simulink model "Demo_V2X_RoadWorks_cs"  (R2014b)
settings: Solver=ode5  SolverMode=SingleTasking  StartTime=0.0  StopTime=18  FixedStep=1/100  RelTol=1e-3
PreLoadFcn:
  | mbxruntime.callbacks.PreLoadFcn(bdroot);
  | check_NUTS_defined;
  | 
  | assignin('base',['model_closed_' bdroot],false);
PostLoadFcn:
  | mbxruntime.callbacks.PostLoadFcn(bdroot);
InitFcn:
  | mbxruntime.callbacks.InitFcn(bdroot);
StartFcn:
  | mbxruntime.callbacks.StartFcn(bdroot);
StopFcn:
  | mbxruntime.callbacks.StopFcn(bdroot);
model workspace: external: MAT-File .\Demo_V2X_RoadWorks_cs_hws.mat (data not in the file)
undefined symbols (not defined in the file or in its folder): InitializeBus, mbxruntime, Newton, Raphson, tabledata
undefined symbols (not defined in the file): Demo_V2X_RoadWorks_cs_002408181c311178, Demo_V2X_RoadWorks_cs_02afd40c5576fd79, Demo_V2X_RoadWorks_cs_09062d95c4976b80, Demo_V2X_RoadWorks_cs_0ad60e46608f1bfe, Demo_V2X_RoadWorks_cs_0b386a01b2cd5e8d, Demo_V2X_RoadWorks_cs_0d795afaa024d2ee, Demo_V2X_RoadWorks_cs_104085e65c337077, Demo_V2X_RoadWorks_cs_126564f7b2997a49, Demo_V2X_RoadWorks_cs_15e6e2595e8bf329, Demo_V2X_RoadWorks_cs_16adfea7655bce18, Demo_V2X_RoadWorks_cs_18ab2686f8449f50, Demo_V2X_RoadWorks_cs_1c28437def32f9f6, Demo_V2X_RoadWorks_cs_1d541c73c3d8f25b, Demo_V2X_RoadWorks_cs_1fb1f994fe012d27, Demo_V2X_RoadWorks_cs_20c117b9827230b9, Demo_V2X_RoadWorks_cs_220b1226a84e3b37, Demo_V2X_RoadWorks_cs_24814049c8ab2e18, Demo_V2X_RoadWorks_cs_24a281220a6492a7, Demo_V2X_RoadWorks_cs_279aea126b4236ad, Demo_V2X_RoadWorks_cs_28eadd0b23e572db, Demo_V2X_RoadWorks_cs_291fe7210f9ba434, Demo_V2X_RoadWorks_cs_2fd90504f8814746, Demo_V2X_RoadWorks_cs_33c1737bfc1c651f, Demo_V2X_RoadWorks_cs_388e22d5b1056b8f, Demo_V2X_RoadWorks_cs_3e3a415e868663e7, Demo_V2X_RoadWorks_cs_45759eb0c1816b1e, Demo_V2X_RoadWorks_cs_45f301cf6c396570, Demo_V2X_RoadWorks_cs_47686124f5151dea, Demo_V2X_RoadWorks_cs_487931e8a8cef1d6, Demo_V2X_RoadWorks_cs_54cb5626dca53ab7, Demo_V2X_RoadWorks_cs_56c0a253fe7e7ec0, Demo_V2X_RoadWorks_cs_5921488c0ba4168e, Demo_V2X_RoadWorks_cs_5ca0c70551eea1b3, Demo_V2X_RoadWorks_cs_5cc6ddb60eb17926, Demo_V2X_RoadWorks_cs_5dda33a127b53dd9, Demo_V2X_RoadWorks_cs_60729aca19e3b8ea, Demo_V2X_RoadWorks_cs_61616eaaf58ec115, Demo_V2X_RoadWorks_cs_63af626c9fae5224, Demo_V2X_RoadWorks_cs_649c6af7b111a61f, Demo_V2X_RoadWorks_cs_64e2df335ac415c1, Demo_V2X_RoadWorks_cs_6530f1ae727e39fe, Demo_V2X_RoadWorks_cs_6837be8d052ff1e3, Demo_V2X_RoadWorks_cs_6e8b51a123f1a201, Demo_V2X_RoadWorks_cs_6f4ec518a68cacb3, Demo_V2X_RoadWorks_cs_74dac4a6b9859226, Demo_V2X_RoadWorks_cs_75671d8cae67d5b6, Demo_V2X_RoadWorks_cs_756d40a88ae84d39, Demo_V2X_RoadWorks_cs_77c7cbc4fa1cdaa5, Demo_V2X_RoadWorks_cs_7b9fbc44403bb8f3, Demo_V2X_RoadWorks_cs_7c118b74c8d14c00, Demo_V2X_RoadWorks_cs_7c4a172761f05beb, Demo_V2X_RoadWorks_cs_80b7a78efe24d5f1, Demo_V2X_RoadWorks_cs_82d65efce1f7c4ea, Demo_V2X_RoadWorks_cs_8be5dc2565229ce9, Demo_V2X_RoadWorks_cs_8dc36f0ab6cec640, Demo_V2X_RoadWorks_cs_91305dd1362bb00d, Demo_V2X_RoadWorks_cs_929c2ffed1faf33f, Demo_V2X_RoadWorks_cs_95615bcbc0d062f1, Demo_V2X_RoadWorks_cs_99a6391a40f894df, Demo_V2X_RoadWorks_cs_9caa19175765ea5d ... (+52)
libraries: PreScanSimulinkLibrary x34, simulink_extras x15, simulink x6
(part 5 of 16)

== system Demo_V2X_RoadWorks_cs/SELF_Male_Regular_BendingOver_1 ==
  Sensor : S-Function  FunctionName=sfun_SelfSensor  Parameters=UniqueID, TimeStep  EnableBusSupport=off  mask(PreScan Source Block: SELF){UniqueID=4029, TimeStep=1/100}
      mask prompts: UniqueID "Auto-Assigned: Unique ID"; TimeStep "Auto-Assigned: Upload Period [s]"
      mask help:
      | The SELF port shows (state) information of the actor itself. The outputs are position in the experiment's axis system and the GPS coordinates, and the object's absolute velocity and compass heading.
      |
      | For more information, please click Help.
      mask Help: eval('openHelp(462)')
      mask Display: image(imread('GPS.png'))
  SELF_Male_Regular_BendingOver_1 : Outport  Tag=outport/SelfPort  OutDataTypeStr=Bus: PRESCAN_SELFSENSORDATA  PortDimensions=1  SampleTime=1/100
  wires:
  Sensor/1 -> SELF_Male_Regular_BendingOver_1/1

== system Demo_V2X_RoadWorks_cs/SELF_Male_Regular_LeaningBack_1 ==
  Sensor : S-Function  FunctionName=sfun_SelfSensor  Parameters=UniqueID, TimeStep  EnableBusSupport=off  mask(PreScan Source Block: SELF){UniqueID=4031, TimeStep=1/100}
      mask prompts: UniqueID "Auto-Assigned: Unique ID"; TimeStep "Auto-Assigned: Upload Period [s]"
      mask help:
      | The SELF port shows (state) information of the actor itself. The outputs are position in the experiment's axis system and the GPS coordinates, and the object's absolute velocity and compass heading.
      |
      | For more information, please click Help.
      mask Help: eval('openHelp(462)')
      mask Display: image(imread('GPS.png'))
  SELF_Male_Regular_LeaningBack_1 : Outport  Tag=outport/SelfPort  OutDataTypeStr=Bus: PRESCAN_SELFSENSORDATA  PortDimensions=1  SampleTime=1/100
  wires:
  Sensor/1 -> SELF_Male_Regular_LeaningBack_1/1

== system Demo_V2X_RoadWorks_cs/SELF_Male_Regular_LeaningBack_2 ==
  Sensor : S-Function  FunctionName=sfun_SelfSensor  Parameters=UniqueID, TimeStep  EnableBusSupport=off  mask(PreScan Source Block: SELF){UniqueID=4032, TimeStep=1/100}
      mask prompts: UniqueID "Auto-Assigned: Unique ID"; TimeStep "Auto-Assigned: Upload Period [s]"
      mask help:
      | The SELF port shows (state) information of the actor itself. The outputs are position in the experiment's axis system and the GPS coordinates, and the object's absolute velocity and compass heading.
      |
      | For more information, please click Help.
      mask Help: eval('openHelp(462)')
      mask Display: image(imread('GPS.png'))
  SELF_Male_Regular_LeaningBack_2 : Outport  Tag=outport/SelfPort  OutDataTypeStr=Bus: PRESCAN_SELFSENSORDATA  PortDimensions=1  SampleTime=1/100
  wires:
  Sensor/1 -> SELF_Male_Regular_LeaningBack_2/1

== system Demo_V2X_RoadWorks_cs/SELF_Male_Regular_Leaning_1 ==
  Sensor : S-Function  FunctionName=sfun_SelfSensor  Parameters=UniqueID, TimeStep  EnableBusSupport=off  mask(PreScan Source Block: SELF){UniqueID=4030, TimeStep=1/100}
      mask prompts: UniqueID "Auto-Assigned: Unique ID"; TimeStep "Auto-Assigned: Upload Period [s]"
      mask help:
      | The SELF port shows (state) information of the actor itself. The outputs are position in the experiment's axis system and the GPS coordinates, and the object's absolute velocity and compass heading.
      |
      | For more information, please click Help.
      mask Help: eval('openHelp(462)')
      mask Display: image(imread('GPS.png'))
  SELF_Male_Regular_Leaning_1 : Outport  Tag=outport/SelfPort  OutDataTypeStr=Bus: PRESCAN_SELFSENSORDATA  PortDimensions=1  SampleTime=1/100
  wires:
  Sensor/1 -> SELF_Male_Regular_Leaning_1/1

== system Demo_V2X_RoadWorks_cs/SELF_Male_Regular_LyingDown_1 ==
  Sensor : S-Function  FunctionName=sfun_SelfSensor  Parameters=UniqueID, TimeStep  EnableBusSupport=off  mask(PreScan Source Block: SELF){UniqueID=4028, TimeStep=1/100}
      mask prompts: UniqueID "Auto-Assigned: Unique ID"; TimeStep "Auto-Assigned: Upload Period [s]"
      mask help:
      | The SELF port shows (state) information of the actor itself. The outputs are position in the experiment's axis system and the GPS coordinates, and the object's absolute velocity and compass heading.
      |
      | For more information, please click Help.
      mask Help: eval('openHelp(462)')
      mask Display: image(imread('GPS.png'))
  SELF_Male_Regular_LyingDown_1 : Outport  Tag=outport/SelfPort  OutDataTypeStr=Bus: PRESCAN_SELFSENSORDATA  PortDimensions=1  SampleTime=1/100
  wires:
  Sensor/1 -> SELF_Male_Regular_LyingDown_1/1

== system Demo_V2X_RoadWorks_cs/SELF_Mazda_RX8_1 ==
  Sensor : S-Function  FunctionName=sfun_SelfSensor  Parameters=UniqueID, TimeStep  EnableBusSupport=off  mask(PreScan Source Block: SELF){UniqueID=3607, TimeStep=1/100}
      mask prompts: UniqueID "Auto-Assigned: Unique ID"; TimeStep "Auto-Assigned: Upload Period [s]"
      mask help:
      | The SELF port shows (state) information of the actor itself. The outputs are position in the experiment's axis system and the GPS coordinates, and the object's absolute velocity and compass heading.
      |
      | For more information, please click Help.
      mask Help: eval('openHelp(462)')
      mask Display: image(imread('GPS.png'))
  SELF_Mazda_RX8_1 : Outport  Tag=outport/SelfPort  OutDataTypeStr=Bus: PRESCAN_SELFSENSORDATA  PortDimensions=1  SampleTime=1/100
  wires:
  Sensor/1 -> SELF_Mazda_RX8_1/1

== system Demo_V2X_RoadWorks_cs/SELF_Nissan_Cabstar_1 ==
  Sensor : S-Function  FunctionName=sfun_SelfSensor  Parameters=UniqueID, TimeStep  EnableBusSupport=off  mask(PreScan Source Block: SELF){UniqueID=3606, TimeStep=1/100}
      mask prompts: UniqueID "Auto-Assigned: Unique ID"; TimeStep "Auto-Assigned: Upload Period [s]"
      mask help:
      | The SELF port shows (state) information of the actor itself. The outputs are position in the experiment's axis system and the GPS coordinates, and the object's absolute velocity and compass heading.
      |
      | For more information, please click Help.
      mask Help: eval('openHelp(462)')
      mask Display: image(imread('GPS.png'))
  SELF_Nissan_Cabstar_1 : Outport  Tag=outport/SelfPort  OutDataTypeStr=Bus: PRESCAN_SELFSENSORDATA  PortDimensions=1  SampleTime=1/100
  wires:
  Sensor/1 -> SELF_Nissan_Cabstar_1/1

== system Demo_V2X_RoadWorks_cs/SELF_Sphere_1 ==
  Sensor : S-Function  FunctionName=sfun_SelfSensor  Parameters=UniqueID, TimeStep  EnableBusSupport=off  mask(PreScan Source Block: SELF){UniqueID=3615, TimeStep=1/100}
      mask prompts: UniqueID "Auto-Assigned: Unique ID"; TimeStep "Auto-Assigned: Upload Period [s]"
      mask help:
      | The SELF port shows (state) information of the actor itself. The outputs are position in the experiment's axis system and the GPS coordinates, and the object's absolute velocity and compass heading.
      |
      | For more information, please click Help.
      mask Help: eval('openHelp(462)')
      mask Display: image(imread('GPS.png'))
  SELF_Sphere_1 : Outport  Tag=outport/SelfPort  OutDataTypeStr=Bus: PRESCAN_SELFSENSORDATA  PortDimensions=1  SampleTime=1/100
  wires:
  Sensor/1 -> SELF_Sphere_1/1

== system Demo_V2X_RoadWorks_cs/SELF_Toyota_Previa_1 ==
  Sensor : S-Function  FunctionName=sfun_SelfSensor  Parameters=UniqueID, TimeStep  EnableBusSupport=off  mask(PreScan Source Block: SELF){UniqueID=3608, TimeStep=1/100}
      mask prompts: UniqueID "Auto-Assigned: Unique ID"; TimeStep "Auto-Assigned: Upload Period [s]"
      mask help:
      | The SELF port shows (state) information of the actor itself. The outputs are position in the experiment's axis system and the GPS coordinates, and the object's absolute velocity and compass heading.
      |
      | For more information, please click Help.
      mask Help: eval('openHelp(462)')
      mask Display: image(imread('GPS.png'))
  SELF_Toyota_Previa_1 : Outport  Tag=outport/SelfPort  OutDataTypeStr=Bus: PRESCAN_SELFSENSORDATA  PortDimensions=1  SampleTime=1/100
  wires:
  Sensor/1 -> SELF_Toyota_Previa_1/1

== system Demo_V2X_RoadWorks_cs/SELF_Toyota_Yaris_1 ==
  Sensor : S-Function  FunctionName=sfun_SelfSensor  Parameters=UniqueID, TimeStep  EnableBusSupport=off  mask(PreScan Source Block: SELF){UniqueID=3534, TimeStep=1/100}
      mask prompts: UniqueID "Auto-Assigned: Unique ID"; TimeStep "Auto-Assigned: Upload Period [s]"
      mask help:
      | The SELF port shows (state) information of the actor itself. The outputs are position in the experiment's axis system and the GPS coordinates, and the object's absolute velocity and compass heading.
      |
      | For more information, please click Help.
      mask Help: eval('openHelp(462)')
      mask Display: image(imread('GPS.png'))
  SELF_Toyota_Yaris_1 : Outport  Tag=outport/SelfPort  OutDataTypeStr=Bus: PRESCAN_SELFSENSORDATA  PortDimensions=1  SampleTime=1/100
  wires:
  Sensor/1 -> SELF_Toyota_Yaris_1/1

== system Demo_V2X_RoadWorks_cs/STATE_Actros_1860_1_bus ==
  STATE_Actros_1860_1_bus : Inport  Tag=inport/StatePort  OutDataTypeStr=Bus: PRESCAN_STATEACTUATORDATA  PortDimensions=1  SampleTime=1/100  BusOutputAsStruct=on
  Actuator : S-Function  FunctionName=sfun_StateActuator  Parameters=UniqueID, TimeStep  EnableBusSupport=off  mask(PreScan Sink Block: State){UniqueID=3711, TimeStep=1/100}
      mask prompts: UniqueID "Auto-Assigned: Unique ID"; TimeStep "Auto-Assigned: Upload Period [s]"
      mask help:
      | The Actor State contains a vector signal of size (9x1), containing the following signals:
      |
      | -  Position    	(x,y,z)             	[m]
      | -  Velocity    	(vx,vy,vz)         	[m/s]
      | -  Angles       	(Roll, Pitch, Yaw)	[rad]
      |
      | The Actor state is defined in the global axis system.
      | The state is superponed on the Initial position defined in the GUI.
      |
      | For more information, please click Help.
      mask Help: eval('openHelp(222)')
      mask Display: image(imread('State.png'))
  wires:
  STATE_Actros_1860_1_bus/1 -> Actuator/1

== system Demo_V2X_RoadWorks_cs/STATE_Actros_2541_1_bus ==
  STATE_Actros_2541_1_bus : Inport  Tag=inport/StatePort  OutDataTypeStr=Bus: PRESCAN_STATEACTUATORDATA  PortDimensions=1  SampleTime=1/100  BusOutputAsStruct=on
  Actuator : S-Function  FunctionName=sfun_StateActuator  Parameters=UniqueID, TimeStep  EnableBusSupport=off  mask(PreScan Sink Block: State){UniqueID=3609, TimeStep=1/100}
      mask prompts: UniqueID "Auto-Assigned: Unique ID"; TimeStep "Auto-Assigned: Upload Period [s]"
      mask help:
      | The Actor State contains a vector signal of size (9x1), containing the following signals:
      |
      | -  Position    	(x,y,z)             	[m]
      | -  Velocity    	(vx,vy,vz)         	[m/s]
      | -  Angles       	(Roll, Pitch, Yaw)	[rad]
      |
      | The Actor state is defined in the global axis system.
      | The state is superponed on the Initial position defined in the GUI.
      |
      | For more information, please click Help.
      mask Help: eval('openHelp(222)')
      mask Display: image(imread('State.png'))
  wires:
  STATE_Actros_2541_1_bus/1 -> Actuator/1

== system Demo_V2X_RoadWorks_cs/STATE_Audi_A8_1_bus ==
  STATE_Audi_A8_1_bus : Inport  Tag=inport/StatePort  OutDataTypeStr=Bus: PRESCAN_STATEACTUATORDATA  PortDimensions=1  SampleTime=1/100  BusOutputAsStruct=on
  Actuator : S-Function  FunctionName=sfun_StateActuator  Parameters=UniqueID, TimeStep  EnableBusSupport=off  mask(PreScan Sink Block: State){UniqueID=1227, TimeStep=1/100}
      mask prompts: UniqueID "Auto-Assigned: Unique ID"; TimeStep "Auto-Assigned: Upload Period [s]"
      mask help:
      | The Actor State contains a vector signal of size (9x1), containing the following signals:
      |
      | -  Position    	(x,y,z)             	[m]
      | -  Velocity    	(vx,vy,vz)         	[m/s]
      | -  Angles       	(Roll, Pitch, Yaw)	[rad]
      |
      | The Actor state is defined in the global axis system.
      | The state is superponed on the Initial position defined in the GUI.
      |
      | For more information, please click Help.
      mask Help: eval('openHelp(222)')
      mask Display: image(imread('State.png'))
  wires:
  STATE_Audi_A8_1_bus/1 -> Actuator/1

== system Demo_V2X_RoadWorks_cs/STATE_BMW_X5_1_bus ==
  STATE_BMW_X5_1_bus : Inport  Tag=inport/StatePort  OutDataTypeStr=Bus: PRESCAN_STATEACTUATORDATA  PortDimensions=1  SampleTime=1/100  BusOutputAsStruct=on
  Actuator : S-Function  FunctionName=sfun_StateActuator  Parameters=UniqueID, TimeStep  EnableBusSupport=off  mask(PreScan Sink Block: State){UniqueID=3531, TimeStep=1/100}
      mask prompts: UniqueID "Auto-Assigned: Unique ID"; TimeStep "Auto-Assigned: Upload Period [s]"
      mask help:
      | The Actor State contains a vector signal of size (9x1), containing the following signals:
      |
      | -  Position    	(x,y,z)             	[m]
      | -  Velocity    	(vx,vy,vz)         	[m/s]
      | -  Angles       	(Roll, Pitch, Yaw)	[rad]
      |
      | The Actor state is defined in the global axis system.
      | The state is superponed on the Initial position defined in the GUI.
      |
      | For more information, please click Help.
      mask Help: eval('openHelp(222)')
      mask Display: image(imread('State.png'))
  wires:
  STATE_BMW_X5_1_bus/1 -> Actuator/1

== system Demo_V2X_RoadWorks_cs/STATE_CarTrailer_SingleAxle_1_bus ==
  STATE_CarTrailer_SingleAxle_1_bus : Inport  Tag=inport/StatePort  OutDataTypeStr=Bus: PRESCAN_STATEACTUATORDATA  PortDimensions=1  SampleTime=1/100  BusOutputAsStruct=on
  Actuator : S-Function  FunctionName=sfun_StateActuator  Parameters=UniqueID, TimeStep  EnableBusSupport=off  mask(PreScan Sink Block: State){UniqueID=4026, TimeStep=1/100}
      mask prompts: UniqueID "Auto-Assigned: Unique ID"; TimeStep "Auto-Assigned: Upload Period [s]"
      mask help:
      | The Actor State contains a vector signal of size (9x1), containing the following signals:
      |
      | -  Position    	(x,y,z)             	[m]
      | -  Velocity    	(vx,vy,vz)         	[m/s]
      | -  Angles       	(Roll, Pitch, Yaw)	[rad]
      |
      | The Actor state is defined in the global axis system.
      | The state is superponed on the Initial position defined in the GUI.
      |
      | For more information, please click Help.
      mask Help: eval('openHelp(222)')
      mask Display: image(imread('State.png'))
  wires:
  STATE_CarTrailer_SingleAxle_1_bus/1 -> Actuator/1

== system Demo_V2X_RoadWorks_cs/STATE_ChessPlaneBox_1_bus ==
  STATE_ChessPlaneBox_1_bus : Inport  Tag=inport/StatePort  OutDataTypeStr=Bus: PRESCAN_STATEACTUATORDATA  PortDimensions=1  SampleTime=1/100  BusOutputAsStruct=on
  Actuator : S-Function  FunctionName=sfun_StateActuator  Parameters=UniqueID, TimeStep  EnableBusSupport=off  mask(PreScan Sink Block: State){UniqueID=4034, TimeStep=1/100}
      mask prompts: UniqueID "Auto-Assigned: Unique ID"; TimeStep "Auto-Assigned: Upload Period [s]"
      mask help:
      | The Actor State contains a vector signal of size (9x1), containing the following signals:
      |
      | -  Position    	(x,y,z)             	[m]
      | -  Velocity    	(vx,vy,vz)         	[m/s]
      | -  Angles       	(Roll, Pitch, Yaw)	[rad]
      |
      | The Actor state is defined in the global axis system.
      | The state is superponed on the Initial position defined in the GUI.
      |
      | For more information, please click Help.
      mask Help: eval('openHelp(222)')
      mask Display: image(imread('State.png'))
  wires:
  STATE_ChessPlaneBox_1_bus/1 -> Actuator/1

== system Demo_V2X_RoadWorks_cs/STATE_Citroen_C3_1_bus ==
  STATE_Citroen_C3_1_bus : Inport  Tag=inport/StatePort  OutDataTypeStr=Bus: PRESCAN_STATEACTUATORDATA  PortDimensions=1  SampleTime=1/100  BusOutputAsStruct=on
  Actuator : S-Function  FunctionName=sfun_StateActuator  Parameters=UniqueID, TimeStep  EnableBusSupport=off  mask(PreScan Sink Block: State){UniqueID=3533, TimeStep=1/100}
      mask prompts: UniqueID "Auto-Assigned: Unique ID"; TimeStep "Auto-Assigned: Upload Period [s]"
      mask help:
      | The Actor State contains a vector signal of size (9x1), containing the following signals:
      |
      | -  Position    	(x,y,z)             	[m]
      | -  Velocity    	(vx,vy,vz)         	[m/s]
      | -  Angles       	(Roll, Pitch, Yaw)	[rad]
      |
      | The Actor state is defined in the global axis system.
      | The state is superponed on the Initial position defined in the GUI.
      |
      | For more information, please click Help.
      mask Help: eval('openHelp(222)')
      mask Display: image(imread('State.png'))
  wires:
  STATE_Citroen_C3_1_bus/1 -> Actuator/1

== system Demo_V2X_RoadWorks_cs/STATE_Fiat_Bravo_1_bus ==
  STATE_Fiat_Bravo_1_bus : Inport  Tag=inport/StatePort  OutDataTypeStr=Bus: PRESCAN_STATEACTUATORDATA  PortDimensions=1  SampleTime=1/100  BusOutputAsStruct=on
  Actuator : S-Function  FunctionName=sfun_StateActuator  Parameters=UniqueID, TimeStep  EnableBusSupport=off  mask(PreScan Sink Block: State){UniqueID=3535, TimeStep=1/100}
      mask prompts: UniqueID "Auto-Assigned: Unique ID"; TimeStep "Auto-Assigned: Upload Period [s]"
      mask help:
      | The Actor State contains a vector signal of size (9x1), containing the following signals:
      |
      | -  Position    	(x,y,z)             	[m]
      | -  Velocity    	(vx,vy,vz)         	[m/s]
      | -  Angles       	(Roll, Pitch, Yaw)	[rad]
      |
      | The Actor state is defined in the global axis system.
      | The state is superponed on the Initial position defined in the GUI.
      |
      | For more information, please click Help.
      mask Help: eval('openHelp(222)')
      mask Display: image(imread('State.png'))
  wires:
  STATE_Fiat_Bravo_1_bus/1 -> Actuator/1

== system Demo_V2X_RoadWorks_cs/STATE_Ford_FocusWagon_1_bus ==
  STATE_Ford_FocusWagon_1_bus : Inport  Tag=inport/StatePort  OutDataTypeStr=Bus: PRESCAN_STATEACTUATORDATA  PortDimensions=1  SampleTime=1/100  BusOutputAsStruct=on
  Actuator : S-Function  FunctionName=sfun_StateActuator  Parameters=UniqueID, TimeStep  EnableBusSupport=off  mask(PreScan Sink Block: State){UniqueID=3532, TimeStep=1/100}
      mask prompts: UniqueID "Auto-Assigned: Unique ID"; TimeStep "Auto-Assigned: Upload Period [s]"
      mask help:
      | The Actor State contains a vector signal of size (9x1), containing the following signals:
      |
      | -  Position    	(x,y,z)             	[m]
      | -  Velocity    	(vx,vy,vz)         	[m/s]
      | -  Angles       	(Roll, Pitch, Yaw)	[rad]
      |
      | The Actor state is defined in the global axis system.
      | The state is superponed on the Initial position defined in the GUI.
      |
      | For more information, please click Help.
      mask Help: eval('openHelp(222)')
      mask Display: image(imread('State.png'))
  wires:
  STATE_Ford_FocusWagon_1_bus/1 -> Actuator/1

== system Demo_V2X_RoadWorks_cs/STATE_Male_Regular_BendingOver_1_bus ==
  STATE_Male_Regular_BendingOver_1_bus : Inport  Tag=inport/StatePort  OutDataTypeStr=Bus: PRESCAN_STATEACTUATORDATA  PortDimensions=1  SampleTime=1/100  BusOutputAsStruct=on
  Actuator : S-Function  FunctionName=sfun_StateActuator  Parameters=UniqueID, TimeStep  EnableBusSupport=off  mask(PreScan Sink Block: State){UniqueID=4029, TimeStep=1/100}
      mask prompts: UniqueID "Auto-Assigned: Unique ID"; TimeStep "Auto-Assigned: Upload Period [s]"
      mask help:
      | The Actor State contains a vector signal of size (9x1), containing the following signals:
      |
      | -  Position    	(x,y,z)             	[m]
      | -  Velocity    	(vx,vy,vz)         	[m/s]
      | -  Angles       	(Roll, Pitch, Yaw)	[rad]
      |
      | The Actor state is defined in the global axis system.
      | The state is superponed on the Initial position defined in the GUI.
      |
      | For more information, please click Help.
      mask Help: eval('openHelp(222)')
      mask Display: image(imread('State.png'))
  wires:
  STATE_Male_Regular_BendingOver_1_bus/1 -> Actuator/1

== system Demo_V2X_RoadWorks_cs/STATE_Male_Regular_LeaningBack_1_bus ==
  STATE_Male_Regular_LeaningBack_1_bus : Inport  Tag=inport/StatePort  OutDataTypeStr=Bus: PRESCAN_STATEACTUATORDATA  PortDimensions=1  SampleTime=1/100  BusOutputAsStruct=on
  Actuator : S-Function  FunctionName=sfun_StateActuator  Parameters=UniqueID, TimeStep  EnableBusSupport=off  mask(PreScan Sink Block: State){UniqueID=4031, TimeStep=1/100}
      mask prompts: UniqueID "Auto-Assigned: Unique ID"; TimeStep "Auto-Assigned: Upload Period [s]"
      mask help:
      | The Actor State contains a vector signal of size (9x1), containing the following signals:
      |
      | -  Position    	(x,y,z)             	[m]
      | -  Velocity    	(vx,vy,vz)         	[m/s]
      | -  Angles       	(Roll, Pitch, Yaw)	[rad]
      |
      | The Actor state is defined in the global axis system.
      | The state is superponed on the Initial position defined in the GUI.
      |
      | For more information, please click Help.
      mask Help: eval('openHelp(222)')
      mask Display: image(imread('State.png'))
  wires:
  STATE_Male_Regular_LeaningBack_1_bus/1 -> Actuator/1

== system Demo_V2X_RoadWorks_cs/STATE_Male_Regular_LeaningBack_2_bus ==
  STATE_Male_Regular_LeaningBack_2_bus : Inport  Tag=inport/StatePort  OutDataTypeStr=Bus: PRESCAN_STATEACTUATORDATA  PortDimensions=1  SampleTime=1/100  BusOutputAsStruct=on
  Actuator : S-Function  FunctionName=sfun_StateActuator  Parameters=UniqueID, TimeStep  EnableBusSupport=off  mask(PreScan Sink Block: State){UniqueID=4032, TimeStep=1/100}
      mask prompts: UniqueID "Auto-Assigned: Unique ID"; TimeStep "Auto-Assigned: Upload Period [s]"
      mask help:
      | The Actor State contains a vector signal of size (9x1), containing the following signals:
      |
      | -  Position    	(x,y,z)             	[m]
      | -  Velocity    	(vx,vy,vz)         	[m/s]
      | -  Angles       	(Roll, Pitch, Yaw)	[rad]
      |
      | The Actor state is defined in the global axis system.
      | The state is superponed on the Initial position defined in the GUI.
      |
      | For more information, please click Help.
      mask Help: eval('openHelp(222)')
      mask Display: image(imread('State.png'))
  wires:
  STATE_Male_Regular_LeaningBack_2_bus/1 -> Actuator/1

== system Demo_V2X_RoadWorks_cs/STATE_Male_Regular_Leaning_1_bus ==
  STATE_Male_Regular_Leaning_1_bus : Inport  Tag=inport/StatePort  OutDataTypeStr=Bus: PRESCAN_STATEACTUATORDATA  PortDimensions=1  SampleTime=1/100  BusOutputAsStruct=on
  Actuator : S-Function  FunctionName=sfun_StateActuator  Parameters=UniqueID, TimeStep  EnableBusSupport=off  mask(PreScan Sink Block: State){UniqueID=4030, TimeStep=1/100}
      mask prompts: UniqueID "Auto-Assigned: Unique ID"; TimeStep "Auto-Assigned: Upload Period [s]"
      mask help:
      | The Actor State contains a vector signal of size (9x1), containing the following signals:
      |
      | -  Position    	(x,y,z)             	[m]
      | -  Velocity    	(vx,vy,vz)         	[m/s]
      | -  Angles       	(Roll, Pitch, Yaw)	[rad]
      |
      | The Actor state is defined in the global axis system.
      | The state is superponed on the Initial position defined in the GUI.
      |
      | For more information, please click Help.
      mask Help: eval('openHelp(222)')
      mask Display: image(imread('State.png'))
  wires:
  STATE_Male_Regular_Leaning_1_bus/1 -> Actuator/1

== system Demo_V2X_RoadWorks_cs/STATE_Male_Regular_LyingDown_1_bus ==
  STATE_Male_Regular_LyingDown_1_bus : Inport  Tag=inport/StatePort  OutDataTypeStr=Bus: PRESCAN_STATEACTUATORDATA  PortDimensions=1  SampleTime=1/100  BusOutputAsStruct=on
  Actuator : S-Function  FunctionName=sfun_StateActuator  Parameters=UniqueID, TimeStep  EnableBusSupport=off  mask(PreScan Sink Block: State){UniqueID=4028, TimeStep=1/100}
      mask prompts: UniqueID "Auto-Assigned: Unique ID"; TimeStep "Auto-Assigned: Upload Period [s]"
      mask help:
      | The Actor State contains a vector signal of size (9x1), containing the following signals:
      |
      | -  Position    	(x,y,z)             	[m]
      | -  Velocity    	(vx,vy,vz)         	[m/s]
      | -  Angles       	(Roll, Pitch, Yaw)	[rad]
      |
      | The Actor state is defined in the global axis system.
      | The state is superponed on the Initial position defined in the GUI.
      |
      | For more information, please click Help.
      mask Help: eval('openHelp(222)')
      mask Display: image(imread('State.png'))
  wires:
  STATE_Male_Regular_LyingDown_1_bus/1 -> Actuator/1

== system Demo_V2X_RoadWorks_cs/STATE_Mazda_RX8_1_bus ==
  STATE_Mazda_RX8_1_bus : Inport  Tag=inport/StatePort  OutDataTypeStr=Bus: PRESCAN_STATEACTUATORDATA  PortDimensions=1  SampleTime=1/100  BusOutputAsStruct=on
  Actuator : S-Function  FunctionName=sfun_StateActuator  Parameters=UniqueID, TimeStep  EnableBusSupport=off  mask(PreScan Sink Block: State){UniqueID=3607, TimeStep=1/100}
      mask prompts: UniqueID "Auto-Assigned: Unique ID"; TimeStep "Auto-Assigned: Upload Period [s]"
      mask help:
      | The Actor State contains a vector signal of size (9x1), containing the following signals:
      |
      | -  Position    	(x,y,z)             	[m]
      | -  Velocity    	(vx,vy,vz)         	[m/s]
      | -  Angles       	(Roll, Pitch, Yaw)	[rad]
      |
      | The Actor state is defined in the global axis system.
      | The state is superponed on the Initial position defined in the GUI.
      |
      | For more information, please click Help.
      mask Help: eval('openHelp(222)')
      mask Display: image(imread('State.png'))
  wires:
  STATE_Mazda_RX8_1_bus/1 -> Actuator/1

== system Demo_V2X_RoadWorks_cs/STATE_Nissan_Cabstar_1_bus ==
  STATE_Nissan_Cabstar_1_bus : Inport  Tag=inport/StatePort  OutDataTypeStr=Bus: PRESCAN_STATEACTUATORDATA  PortDimensions=1  SampleTime=1/100  BusOutputAsStruct=on
  Actuator : S-Function  FunctionName=sfun_StateActuator  Parameters=UniqueID, TimeStep  EnableBusSupport=off  mask(PreScan Sink Block: State){UniqueID=3606, TimeStep=1/100}
      mask prompts: UniqueID "Auto-Assigned: Unique ID"; TimeStep "Auto-Assigned: Upload Period [s]"
      mask help:
      | The Actor State contains a vector signal of size (9x1), containing the following signals:
      |
      | -  Position    	(x,y,z)             	[m]
      | -  Velocity    	(vx,vy,vz)         	[m/s]
      | -  Angles       	(Roll, Pitch, Yaw)	[rad]
      |
      | The Actor state is defined in the global axis system.
      | The state is superponed on the Initial position defined in the GUI.
      |
      | For more information, please click Help.
      mask Help: eval('openHelp(222)')
      mask Display: image(imread('State.png'))
  wires:
  STATE_Nissan_Cabstar_1_bus/1 -> Actuator/1

== system Demo_V2X_RoadWorks_cs/STATE_Sphere_1_bus ==
  STATE_Sphere_1_bus : Inport  Tag=inport/StatePort  OutDataTypeStr=Bus: PRESCAN_STATEACTUATORDATA  PortDimensions=1  SampleTime=1/100  BusOutputAsStruct=on
  Actuator : S-Function  FunctionName=sfun_StateActuator  Parameters=UniqueID, TimeStep  EnableBusSupport=off  mask(PreScan Sink Block: State){UniqueID=3615, TimeStep=1/100}
      mask prompts: UniqueID "Auto-Assigned: Unique ID"; TimeStep "Auto-Assigned: Upload Period [s]"
      mask help:
      | The Actor State contains a vector signal of size (9x1), containing the following signals:
      |
      | -  Position    	(x,y,z)             	[m]
      | -  Velocity    	(vx,vy,vz)         	[m/s]
      | -  Angles       	(Roll, Pitch, Yaw)	[rad]
      |
      | The Actor state is defined in the global axis system.
      | The state is superponed on the Initial position defined in the GUI.
      |
      | For more information, please click Help.
      mask Help: eval('openHelp(222)')
      mask Display: image(imread('State.png'))
  wires:
  STATE_Sphere_1_bus/1 -> Actuator/1

== system Demo_V2X_RoadWorks_cs/STATE_Toyota_Previa_1_bus ==
  STATE_Toyota_Previa_1_bus : Inport  Tag=inport/StatePort  OutDataTypeStr=Bus: PRESCAN_STATEACTUATORDATA  PortDimensions=1  SampleTime=1/100  BusOutputAsStruct=on
  Actuator : S-Function  FunctionName=sfun_StateActuator  Parameters=UniqueID, TimeStep  EnableBusSupport=off  mask(PreScan Sink Block: State){UniqueID=3608, TimeStep=1/100}
      mask prompts: UniqueID "Auto-Assigned: Unique ID"; TimeStep "Auto-Assigned: Upload Period [s]"
      mask help:
      | The Actor State contains a vector signal of size (9x1), containing the following signals:
      |
      | -  Position    	(x,y,z)             	[m]
      | -  Velocity    	(vx,vy,vz)         	[m/s]
      | -  Angles       	(Roll, Pitch, Yaw)	[rad]
      |
      | The Actor state is defined in the global axis system.
      | The state is superponed on the Initial position defined in the GUI.
      |
      | For more information, please click Help.
      mask Help: eval('openHelp(222)')
      mask Display: image(imread('State.png'))
  wires:
  STATE_Toyota_Previa_1_bus/1 -> Actuator/1

== system Demo_V2X_RoadWorks_cs/STATE_Toyota_Yaris_1_bus ==
  STATE_Toyota_Yaris_1_bus : Inport  Tag=inport/StatePort  OutDataTypeStr=Bus: PRESCAN_STATEACTUATORDATA  PortDimensions=1  SampleTime=1/100  BusOutputAsStruct=on
  Actuator : S-Function  FunctionName=sfun_StateActuator  Parameters=UniqueID, TimeStep  EnableBusSupport=off  mask(PreScan Sink Block: State){UniqueID=3534, TimeStep=1/100}
      mask prompts: UniqueID "Auto-Assigned: Unique ID"; TimeStep "Auto-Assigned: Upload Period [s]"
      mask help:
      | The Actor State contains a vector signal of size (9x1), containing the following signals:
      |
      | -  Position    	(x,y,z)             	[m]
      | -  Velocity    	(vx,vy,vz)         	[m/s]
      | -  Angles       	(Roll, Pitch, Yaw)	[rad]
      |
      | The Actor state is defined in the global axis system.
      | The state is superponed on the Initial position defined in the GUI.
      |
      | For more information, please click Help.
      mask Help: eval('openHelp(222)')
      mask Display: image(imread('State.png'))
  wires:
  STATE_Toyota_Yaris_1_bus/1 -> Actuator/1

== system Demo_V2X_RoadWorks_cs/ScenarioEngine ==
  Clock : Clock
  sfun_ScenarioEngine : S-Function  FunctionName=sfun_ScenarioEngine  Parameters=TimeStep  EnableBusSupport=off
  wires:
  Clock/1 -> sfun_ScenarioEngine/1

== system Demo_V2X_RoadWorks_cs/Sphere_1 ==
  SELF_Sphere_1 : Inport  Tag=inport/SelfPort  OutDataTypeStr=Bus: PRESCAN_SELFSENSORDATA  PortDimensions=1  SampleTime=1/100  BusOutputAsStruct=on
  Dynamics_Empty : Subsystem  Tag=Dynamics_Empty
      mask Help: eval('openHelp(202)')
      mask Display: port_label('output', 1, 'State');text(0,0,' Empty\n')
  SELF_Demux : Subsystem  Tag=demux/SelfPort  mask(PreScan Demux Block:){}
      mask help:
      | The SELF port shows (state) information of the actor itself. The outputs are position in the experiment's axis system and the GPS coordinates, and the object's absolute velocity and compass heading.
      |
      | For more information, please click Help.
      settings: DeleteFcn=PreScanBlockDeleteFcn;
      mask Help: eval('openHelp(462)')
      mask Display:
      | port_label('output',1,'x [m]')
      | port_label('output',2,'y [m]')
      | port_label('output',3,'z [m]','texmode','on')
      | port_label('output',4,'Rotx [deg]','texmode','on')
      | port_label('output',5,'Roty [deg]','texmode','on')
      | port_label('output',6,'Rotz [deg]','texmode','on')
      | port_label('output',7,'GPS lat [deg]','texmode','on')
      | port_label('output',8,'GPS long [deg]','texmode','on')
      | port_label('output',9,'GPS alt [m]','texmode','on')
      | port_label('output',10,'Velocity [m/s]')
      | port_label('output',11,'Heading [deg]')
      | port_label('output',12,'Yaw rate [deg/s]')
  STATE_Sphere_1_rc : RateTransition  Tag=mux_rc/StatePort  OutPortSampleTimeOpt=Inherit
  Terminator_{1..13} (13 alike) : Terminator
  STATE_Sphere_1_bus : Outport  Tag=outport/StatePort  OutDataTypeStr=Bus: PRESCAN_STATEACTUATORDATA  PortDimensions=1  SampleTime=1/100
  wires:
  [state] -> STATE_Sphere_1_rc/1
  SELF_Sphere_1/1 -> SELF_Demux/1(SELF)
  STATE_Sphere_1_rc/1 -> STATE_Sphere_1_bus/1
  Dynamics_Empty/1(State) -> Terminator_1/1
  SELF_Demux/1(x [m]) -> Terminator_2/1
  SELF_Demux/2(y [m]) -> Terminator_3/1
  SELF_Demux/3(z [m]) -> Terminator_4/1
  SELF_Demux/4(rotx [deg]) -> Terminator_5/1
  SELF_Demux/5(roty [deg]) -> Terminator_6/1
  SELF_Demux/6(rotz [deg]) -> Terminator_7/1
  SELF_Demux/7(GPS lat [deg]) -> Terminator_8/1
  SELF_Demux/8(GPS long [deg]) -> Terminator_9/1
  SELF_Demux/9(GPS alt [m]) -> Terminator_10/1
  SELF_Demux/10(velocity [m/s]) -> Terminator_11/1
  SELF_Demux/11(heading [deg]) -> Terminator_12/1
  SELF_Demux/12(yaw rate [deg/s]) -> Terminator_13/1

== system Demo_V2X_RoadWorks_cs/SteeringColumn_pivot_Audi_A8_1 ==
  SteeringColumn_pivot_Audi_A8_1 : Inport  Tag=inport/JointActuator  OutDataTypeStr=Bus: PRESCAN_POSE_DATA  SampleTime=1/100  BusOutputAsStruct=on
  Actuator : Subsystem  Tag=VisuJoint  mask(PreScan Sink Block: VisuJoint){UniqueID=1227, Translate_ObjectID3D=Audi_A8_1.SteeringColumn_pivot, Rotate_ObjectID3D=Audi_A8_1.SteeringColumn_pivot, TimeStep=1/100, DisplayName=[]}
      mask prompts: UniqueID "Parent Unique ID"; Translate_ObjectID3D "Translate Object Name"; Rotate_ObjectID3D "Rotate Object Name"; TimeStep "Simulation Step"; DisplayName "Display Name"
      mask help:
      | The VisuJoint block provides a way to adapt the location and orientation of a part of an object.
      |
      | For more information, please click Help.
      settings: DeleteFcn=PreScanBlockDeleteFcn;
      mask Help: eval('openHelp(223)')
      mask Display: image(imread('Joint.png'))
  wires:
  SteeringColumn_pivot_Audi_A8_1/1 -> Actuator/1(Joint)

== system Demo_V2X_RoadWorks_cs/SteeringWheel_pivot_Audi_A8_1 ==
  SteeringWheel_pivot_Audi_A8_1 : Inport  Tag=inport/JointActuator  OutDataTypeStr=Bus: PRESCAN_POSE_DATA  SampleTime=1/100  BusOutputAsStruct=on
  Actuator : Subsystem  Tag=VisuJoint  mask(PreScan Sink Block: VisuJoint){UniqueID=1227, Translate_ObjectID3D=Audi_A8_1.SteeringWheel_pivot, Rotate_ObjectID3D=Audi_A8_1.SteeringWheel_pivot, TimeStep=1/100, DisplayName=[]}
      mask prompts: UniqueID "Parent Unique ID"; Translate_ObjectID3D "Translate Object Name"; Rotate_ObjectID3D "Rotate Object Name"; TimeStep "Simulation Step"; DisplayName "Display Name"
      mask help:
      | The VisuJoint block provides a way to adapt the location and orientation of a part of an object.
      |
      | For more information, please click Help.
      settings: DeleteFcn=PreScanBlockDeleteFcn;
      mask Help: eval('openHelp(223)')
      mask Display: image(imread('Joint.png'))
  wires:
  SteeringWheel_pivot_Audi_A8_1/1 -> Actuator/1(Joint)

== system Demo_V2X_RoadWorks_cs/Synchronizer ==
  Bus Selector1 : BusSelector  OutputSignals=FederateStopped
  Stop Simulation : Stop
  sfun_Synchronizer : S-Function  FunctionName=sfun_Synchronizer  Parameters=SampleTime  EnableBusSupport=off  mask(Legacy Function){SFunctionSpec=void prescan_synchronizer_outputFcn(void ** work1, PRESCAN_SYNCHRONIZEDATA y1[1]), SampleTime=TimeStep, ShowSpec=on}
      mask prompts: SampleTime "Sample time (-1 for inherited):"; ShowSpec "Display function specification"
      mask help:
      | This block allows you to call the legacy functions specified by the following Legacy Code Tool definition:
      | def.SFunctionName = 'sfun_Synchronizer';
      | def.OutputFcnSpec = 'void prescan_synchronizer_outputFcn(void ** work1, PRESCAN_SYNCHRONIZEDATA y1[1])';
      | def.StartFcnSpec = 'void prescan_synchronizer_startFcn(void ** work1)';
      | def.TerminateFcnSpec = 'void prescan_synchronizer_terminateFcn(void ** work1)';
      | def.HeaderFiles = {'prescan_synchronizer_data.h'};
      | def.HostLibFiles = {'sensorinterfaced.lib'};
      | def.IncPaths = {'src', 'C:\prescandev\vislibrary\vis\..\pimp\include\sensors\InterfaceRTW'};
      | def.SrcPaths = {'src'};
      | def.LibPaths = {'C:\\prescandev\\vislibrary_build\lib'};
      | def.SampleTime = 'parameterized';
      | def.Options.language = 'C';
      mask Help: <p>This block was generated automatically by the Legacy Code Tool. For detailed help on this tool, call<a href="matlab:legacy_code('help')"> legacy_code('help')</a>.</p>
      mask Callback ShowSpec:
      | if strcmp(get_param(gcbh, 'ShowSpec'), 'on')
      |   set_param(gcbh, 'MaskDisplay', sprintf('fprintf(''%s'');', get_param(gcbh, 'SFunctionSpec')));
      | else
      |   set_param(gcbh, 'MaskDisplay', sprintf('fprintf(''%s'');', get_param(gcbh, 'FunctionName')));
      | end
      mask Display: fprintf('void prescan_synchronizer_outputFcn(void ** work1, PRESCAN_SYNCHRONIZEDATA y1[1])');
  wires:
  Bus Selector1/1 -> Stop Simulation/1  "<FederateStopped>"
  sfun_Synchronizer/1 -> Bus Selector1/1

== system Demo_V2X_RoadWorks_cs/Toyota_Previa_1 ==
  SELF_Toyota_Previa_1 : Inport  Tag=inport/SelfPort  OutDataTypeStr=Bus: PRESCAN_SELFSENSORDATA  PortDimensions=1  SampleTime=1/100  BusOutputAsStruct=on
  Dynamics_Empty : Subsystem  Tag=Dynamics_Empty
      mask Help: eval('openHelp(202)')
      mask Display: port_label('output', 1, 'State');text(0,0,' Empty\n')
  Ground_1 : Ground
  Ground_2 : Ground
  SELF_Demux : Subsystem  Tag=demux/SelfPort  mask(PreScan Demux Block:){}
      mask help:
      | The SELF port shows (state) information of the actor itself. The outputs are position in the experiment's axis system and the GPS coordinates, and the object's absolute velocity and compass heading.
      |
      | For more information, please click Help.
      settings: DeleteFcn=PreScanBlockDeleteFcn;
      mask Help: eval('openHelp(462)')
      mask Display:
      | port_label('output',1,'x [m]')
      | port_label('output',2,'y [m]')
      | port_label('output',3,'z [m]','texmode','on')
      | port_label('output',4,'Rotx [deg]','texmode','on')
      | port_label('output',5,'Roty [deg]','texmode','on')
      | port_label('output',6,'Rotz [deg]','texmode','on')
      | port_label('output',7,'GPS lat [deg]','texmode','on')
      | port_label('output',8,'GPS long [deg]','texmode','on')
      | port_label('output',9,'GPS alt [m]','texmode','on')
      | port_label('output',10,'Velocity [m/s]')
      | port_label('output',11,'Heading [deg]')
      | port_label('output',12,'Yaw rate [deg/s]')
  STATE_Toyota_Previa_1_rc : RateTransition  Tag=mux_rc/StatePort  OutPortSampleTimeOpt=Inherit
  Terminator_{1..12} (12 alike) : Terminator
  V2X_6200_CAM_Create : MATLAB Function  LoadFcn=InitializeBus('CAM')  TreatAsAtomicUnit=on
  V2X_6200_DENM_Create : MATLAB Function  LoadFcn=InitializeBus('DENM')  TreatAsAtomicUnit=on
  STATE_Toyota_Previa_1_bus : Outport  Tag=outport/StatePort  OutDataTypeStr=Bus: PRESCAN_STATEACTUATORDATA  PortDimensions=1  SampleTime=1/100
  V2X_Tx6200_CAM_Transmitter : Outport  Tag=outport/plugin/sfun_V2X_CAM_Transmitter  Port=2
  V2X_Tx6200_DENM_Transmitter : Outport  Tag=outport/plugin/sfun_V2X_DENM_Transmitter  Port=3
  wires:
  SELF_Toyota_Previa_1/1 -> SELF_Demux/1(SELF)
  Dynamics_Empty/1(State) -> STATE_Toyota_Previa_1_rc/1
  STATE_Toyota_Previa_1_rc/1 -> STATE_Toyota_Previa_1_bus/1
  V2X_6200_CAM_Create/1(message) -> V2X_Tx6200_CAM_Transmitter/1
  V2X_6200_DENM_Create/1(message) -> V2X_Tx6200_DENM_Transmitter/1
  SELF_Demux/1(x [m]) -> Terminator_1/1
  SELF_Demux/2(y [m]) -> Terminator_2/1
  SELF_Demux/3(z [m]) -> Terminator_3/1
  SELF_Demux/4(rotx [deg]) -> Terminator_4/1
  SELF_Demux/5(roty [deg]) -> Terminator_5/1
  SELF_Demux/6(rotz [deg]) -> Terminator_6/1
  SELF_Demux/7(GPS lat [deg]) -> Terminator_7/1
  SELF_Demux/8(GPS long [deg]) -> Terminator_8/1
  SELF_Demux/9(GPS alt [m]) -> Terminator_9/1
  SELF_Demux/10(velocity [m/s]) -> Terminator_10/1
  SELF_Demux/11(heading [deg]) -> Terminator_11/1
  SELF_Demux/12(yaw rate [deg/s]) -> Terminator_12/1
  Ground_1/1 -> V2X_6200_CAM_Create/1(z)
  Ground_2/1 -> V2X_6200_DENM_Create/1(z)

== system Demo_V2X_RoadWorks_cs/Toyota_Yaris_1 ==
  SELF_Toyota_Yaris_1 : Inport  Tag=inport/SelfPort  OutDataTypeStr=Bus: PRESCAN_SELFSENSORDATA  PortDimensions=1  SampleTime=1/100  BusOutputAsStruct=on
  Dynamics_Empty : Subsystem  Tag=Dynamics_Empty
      mask Help: eval('openHelp(202)')
      mask Display: port_label('output', 1, 'State');text(0,0,' Empty\n')
  Ground_1 : Ground
  Ground_2 : Ground
  SELF_Demux : Subsystem  Tag=demux/SelfPort  mask(PreScan Demux Block:){}
      mask help:
      | The SELF port shows (state) information of the actor itself. The outputs are position in the experiment's axis system and the GPS coordinates, and the object's absolute velocity and compass heading.
      |
      | For more information, please click Help.
      settings: DeleteFcn=PreScanBlockDeleteFcn;
      mask Help: eval('openHelp(462)')
      mask Display:
      | port_label('output',1,'x [m]')
      | port_label('output',2,'y [m]')
      | port_label('output',3,'z [m]','texmode','on')
      | port_label('output',4,'Rotx [deg]','texmode','on')
      | port_label('output',5,'Roty [deg]','texmode','on')
      | port_label('output',6,'Rotz [deg]','texmode','on')
      | port_label('output',7,'GPS lat [deg]','texmode','on')
      | port_label('output',8,'GPS long [deg]','texmode','on')
      | port_label('output',9,'GPS alt [m]','texmode','on')
      | port_label('output',10,'Velocity [m/s]')
      | port_label('output',11,'Heading [deg]')
      | port_label('output',12,'Yaw rate [deg/s]')
  STATE_Toyota_Yaris_1_rc : RateTransition  Tag=mux_rc/StatePort  OutPortSampleTimeOpt=Inherit
  Terminator_{1..12} (12 alike) : Terminator
  V2X_6196_CAM_Create : MATLAB Function  LoadFcn=InitializeBus('CAM')  TreatAsAtomicUnit=on
  V2X_6196_DENM_Create : MATLAB Function  LoadFcn=InitializeBus('DENM')  TreatAsAtomicUnit=on
  STATE_Toyota_Yaris_1_bus : Outport  Tag=outport/StatePort  OutDataTypeStr=Bus: PRESCAN_STATEACTUATORDATA  PortDimensions=1  SampleTime=1/100
  V2X_Tx6196_CAM_Transmitter : Outport  Tag=outport/plugin/sfun_V2X_CAM_Transmitter  Port=2
  V2X_Tx6196_DENM_Transmitter : Outport  Tag=outport/plugin/sfun_V2X_DENM_Transmitter  Port=3
  wires:
  SELF_Toyota_Yaris_1/1 -> SELF_Demux/1(SELF)
  Dynamics_Empty/1(State) -> STATE_Toyota_Yaris_1_rc/1
  STATE_Toyota_Yaris_1_rc/1 -> STATE_Toyota_Yaris_1_bus/1
  V2X_6196_CAM_Create/1(message) -> V2X_Tx6196_CAM_Transmitter/1
  V2X_6196_DENM_Create/1(message) -> V2X_Tx6196_DENM_Transmitter/1
  SELF_Demux/1(x [m]) -> Terminator_1/1
  SELF_Demux/2(y [m]) -> Terminator_2/1
  SELF_Demux/3(z [m]) -> Terminator_3/1
  SELF_Demux/4(rotx [deg]) -> Terminator_4/1
  SELF_Demux/5(roty [deg]) -> Terminator_5/1
  SELF_Demux/6(rotz [deg]) -> Terminator_6/1
  SELF_Demux/7(GPS lat [deg]) -> Terminator_7/1
  SELF_Demux/8(GPS long [deg]) -> Terminator_8/1
  SELF_Demux/9(GPS alt [m]) -> Terminator_9/1
  SELF_Demux/10(velocity [m/s]) -> Terminator_10/1
  SELF_Demux/11(heading [deg]) -> Terminator_11/1
  SELF_Demux/12(yaw rate [deg/s]) -> Terminator_12/1
  Ground_1/1 -> V2X_6196_CAM_Create/1(z)
  Ground_2/1 -> V2X_6196_DENM_Create/1(z)

== system Demo_V2X_RoadWorks_cs/V2X_Rx6115_CAM_Receiver ==
  Sensor : S-Function  LoadFcn=InitializeBus('CAM')  FunctionName=sfun_V2X_CAM_Receiver  Parameters=sensorID, parentID, maxMessages, timestep  EnableBusSupport=off  mask(V2X CAM Receiver Block){sensorID=6115, parentID=1227, maxMessages=11, timestep=1/100}
      mask prompts: sensorID "Receiver ID"; parentID "Parent ID"; maxMessages "Maximum number of messages"; timestep "MATLAB timestep:"
      mask help: V2X Block receiving a CAM message
      mask Display: image(imread('V2XR_grayscale.png'))
  V2X_Rx6115_CAM_Receiver : Outport  Tag=outport/plugin/sfun_V2X_CAM_Receiver
  wires:
  Sensor/1 -> V2X_Rx6115_CAM_Receiver/1

== system Demo_V2X_RoadWorks_cs/V2X_Rx6115_DENM_Receiver ==
  Sensor : S-Function  LoadFcn=InitializeBus('DENM')  FunctionName=sfun_V2X_DENM_Receiver  Parameters=sensorID, parentID, maxMessages, timestep  EnableBusSupport=off  mask(V2X DENM Receiver Block){sensorID=6115, parentID=1227, maxMessages=11, timestep=1/100}
      mask prompts: sensorID "Receiver ID"; parentID "Parent ID"; maxMessages "Maximum number of messages"; timestep "MATLAB timestep:"
      mask help: V2X Block receiving a DENM message
      mask Display: image(imread('V2XR_grayscale.png'))
  V2X_Rx6115_DENM_Receiver : Outport  Tag=outport/plugin/sfun_V2X_DENM_Receiver
  wires:
  Sensor/1 -> V2X_Rx6115_DENM_Receiver/1

== system Demo_V2X_RoadWorks_cs/V2X_Tx6114_CAM_Transmitter ==
  V2X_Tx6114_CAM_Transmitter : Inport  Tag=inport/plugin/sfun_V2X_CAM_Transmitter  BusOutputAsStruct=on
  Actuator : S-Function  FunctionName=sfun_V2X_CAM_Transmitter  Parameters=sensorID, parentID, timestep  EnableBusSupport=off  mask(V2X CAM Transmitter Block){sensorID=6114, parentID=4026, timestep=1/100}
      mask prompts: sensorID "Transmitter ID"; parentID "Parent ID"; timestep "MATLAB timestep:"
      mask help: V2X Block transmitting a CAM message
      mask Display: image(imread('V2XT_grayscale.png'))
  wires:
  V2X_Tx6114_CAM_Transmitter/1 -> Actuator/1

== system Demo_V2X_RoadWorks_cs/V2X_Tx6114_DENM_Transmitter ==
  V2X_Tx6114_DENM_Transmitter : Inport  Tag=inport/plugin/sfun_V2X_DENM_Transmitter  BusOutputAsStruct=on
  Actuator : S-Function  FunctionName=sfun_V2X_DENM_Transmitter  Parameters=sensorID, parentID, timestep  EnableBusSupport=off  mask(V2X DENM Transmitter Block){sensorID=6114, parentID=4026, timestep=1/100}
      mask prompts: sensorID "Transmitter ID"; parentID "Parent ID"; timestep "MATLAB timestep:"
      mask help: V2X Block transmitting a DENM message
      mask Display: image(imread('V2XT_grayscale.png'))
  wires:
  V2X_Tx6114_DENM_Transmitter/1 -> Actuator/1

== system Demo_V2X_RoadWorks_cs/V2X_Tx6193_CAM_Transmitter ==
  V2X_Tx6193_CAM_Transmitter : Inport  Tag=inport/plugin/sfun_V2X_CAM_Transmitter  BusOutputAsStruct=on
  Actuator : S-Function  FunctionName=sfun_V2X_CAM_Transmitter  Parameters=sensorID, parentID, timestep  EnableBusSupport=off  mask(V2X CAM Transmitter Block){sensorID=6193, parentID=3531, timestep=1/100}
      mask prompts: sensorID "Transmitter ID"; parentID "Parent ID"; timestep "MATLAB timestep:"
      mask help: V2X Block transmitting a CAM message
      mask Display: image(imread('V2XT_grayscale.png'))
  wires:
  V2X_Tx6193_CAM_Transmitter/1 -> Actuator/1

== system Demo_V2X_RoadWorks_cs/V2X_Tx6193_DENM_Transmitter ==
  V2X_Tx6193_DENM_Transmitter : Inport  Tag=inport/plugin/sfun_V2X_DENM_Transmitter  BusOutputAsStruct=on
  Actuator : S-Function  FunctionName=sfun_V2X_DENM_Transmitter  Parameters=sensorID, parentID, timestep  EnableBusSupport=off  mask(V2X DENM Transmitter Block){sensorID=6193, parentID=3531, timestep=1/100}
      mask prompts: sensorID "Transmitter ID"; parentID "Parent ID"; timestep "MATLAB timestep:"
      mask help: V2X Block transmitting a DENM message
      mask Display: image(imread('V2XT_grayscale.png'))
  wires:
  V2X_Tx6193_DENM_Transmitter/1 -> Actuator/1

== system Demo_V2X_RoadWorks_cs/V2X_Tx6194_CAM_Transmitter ==
  V2X_Tx6194_CAM_Transmitter : Inport  Tag=inport/plugin/sfun_V2X_CAM_Transmitter  BusOutputAsStruct=on
  Actuator : S-Function  FunctionName=sfun_V2X_CAM_Transmitter  Parameters=sensorID, parentID, timestep  EnableBusSupport=off  mask(V2X CAM Transmitter Block){sensorID=6194, parentID=3532, timestep=1/100}
      mask prompts: sensorID "Transmitter ID"; parentID "Parent ID"; timestep "MATLAB timestep:"
      mask help: V2X Block transmitting a CAM message
      mask Display: image(imread('V2XT_grayscale.png'))
  wires:
  V2X_Tx6194_CAM_Transmitter/1 -> Actuator/1

== system Demo_V2X_RoadWorks_cs/V2X_Tx6194_DENM_Transmitter ==
  V2X_Tx6194_DENM_Transmitter : Inport  Tag=inport/plugin/sfun_V2X_DENM_Transmitter  BusOutputAsStruct=on
  Actuator : S-Function  FunctionName=sfun_V2X_DENM_Transmitter  Parameters=sensorID, parentID, timestep  EnableBusSupport=off  mask(V2X DENM Transmitter Block){sensorID=6194, parentID=3532, timestep=1/100}
      mask prompts: sensorID "Transmitter ID"; parentID "Parent ID"; timestep "MATLAB timestep:"
      mask help: V2X Block transmitting a DENM message
      mask Display: image(imread('V2XT_grayscale.png'))
  wires:
  V2X_Tx6194_DENM_Transmitter/1 -> Actuator/1

== system Demo_V2X_RoadWorks_cs/V2X_Tx6195_CAM_Transmitter ==
  V2X_Tx6195_CAM_Transmitter : Inport  Tag=inport/plugin/sfun_V2X_CAM_Transmitter  BusOutputAsStruct=on
  Actuator : S-Function  FunctionName=sfun_V2X_CAM_Transmitter  Parameters=sensorID, parentID, timestep  EnableBusSupport=off  mask(V2X CAM Transmitter Block){sensorID=6195, parentID=3533, timestep=1/100}
      mask prompts: sensorID "Transmitter ID"; parentID "Parent ID"; timestep "MATLAB timestep:"
      mask help: V2X Block transmitting a CAM message
      mask Display: image(imread('V2XT_grayscale.png'))
  wires:
  V2X_Tx6195_CAM_Transmitter/1 -> Actuator/1

== system Demo_V2X_RoadWorks_cs/V2X_Tx6195_DENM_Transmitter ==
  V2X_Tx6195_DENM_Transmitter : Inport  Tag=inport/plugin/sfun_V2X_DENM_Transmitter  BusOutputAsStruct=on
  Actuator : S-Function  FunctionName=sfun_V2X_DENM_Transmitter  Parameters=sensorID, parentID, timestep  EnableBusSupport=off  mask(V2X DENM Transmitter Block){sensorID=6195, parentID=3533, timestep=1/100}
      mask prompts: sensorID "Transmitter ID"; parentID "Parent ID"; timestep "MATLAB timestep:"
      mask help: V2X Block transmitting a DENM message
      mask Display: image(imread('V2XT_grayscale.png'))
  wires:
  V2X_Tx6195_DENM_Transmitter/1 -> Actuator/1

== system Demo_V2X_RoadWorks_cs/V2X_Tx6196_CAM_Transmitter ==
  V2X_Tx6196_CAM_Transmitter : Inport  Tag=inport/plugin/sfun_V2X_CAM_Transmitter  BusOutputAsStruct=on
  Actuator : S-Function  FunctionName=sfun_V2X_CAM_Transmitter  Parameters=sensorID, parentID, timestep  EnableBusSupport=off  mask(V2X CAM Transmitter Block){sensorID=6196, parentID=3534, timestep=1/100}
      mask prompts: sensorID "Transmitter ID"; parentID "Parent ID"; timestep "MATLAB timestep:"
      mask help: V2X Block transmitting a CAM message
      mask Display: image(imread('V2XT_grayscale.png'))
  wires:
  V2X_Tx6196_CAM_Transmitter/1 -> Actuator/1
